simulink model "px4demo_mavlink_rc"  (R2017b)
settings: Solver=FixedStepDiscrete  StartTime=0.0  StopTime=inf  RelTol=1e-3  EnableMultiTasking=on
undefined symbols (not defined in the file or in its folder): RC_INPUT_SOURCE_ENUM, RGBLED_COLOR_ENUM, RGBLED_MODE_ENUM
libraries: pixhawk_slib_sensors_actuators x2, simulink x1, pixhawk_slib_uORB_RW x1
Description:
  | PX4 PSP Demo Model publishing a MAVLINK status text message
  | 
  | Example model for using MAVLINK in Simulink
settings Model: Creator=skuznick  LastModifiedBy=skuznick
settings SolverCC: PositivePriorityOrder=on
settings OptimizationCC: DefaultParameterBehavior=Inlined  PassReuseOutputArgsAs=Individual arguments  MaxStackSize=64
settings DebuggingCC: ParameterTunabilityLossMsg=error
settings HardwareCC: ProdBitPerPointer=32  ProdBitPerSizeT=32  ProdBitPerPtrDiffT=32  ProdLargestAtomicInteger=Long  ProdLargestAtomicFloat=Double  ProdWordSize=32  ProdHWDeviceType=ARM Compatible->ARM Cortex
settings SFSimCC: MATLABDynamicMemAlloc=off
settings RTWCC: SystemTargetFile=ert.tlc  HardwareBoard=Pixhawk PX4  TemplateMakefile=ert_default_tmf  GenerateReport=on  Toolchain=Pixhawk Toolchain  BuildConfiguration=Faster Runs  IncludeHyperlinkInReport=on  LaunchReport=on  GenerateTraceInfo=on  GenerateTraceReport=on  GenerateTraceReportSl=on  GenerateTraceReportSf=on  GenerateTraceReportEml=on
settings CodeAppCC: ForceParamTrailComments=on  IgnoreCustomStorageClasses=off  OperatorAnnotations=on  SimulinkDataObjDesc=on  SFDataObjDesc=on  MATLABFcnDesc=on  InsertBlockDesc=on  StateflowObjectComments=on  MATLABSourceComments=on
settings ERTTargetCC: InlinedParameterPlacement=NonHierarchical  ERTCustomFileTemplate=px4_codertarget_file_process.tlc

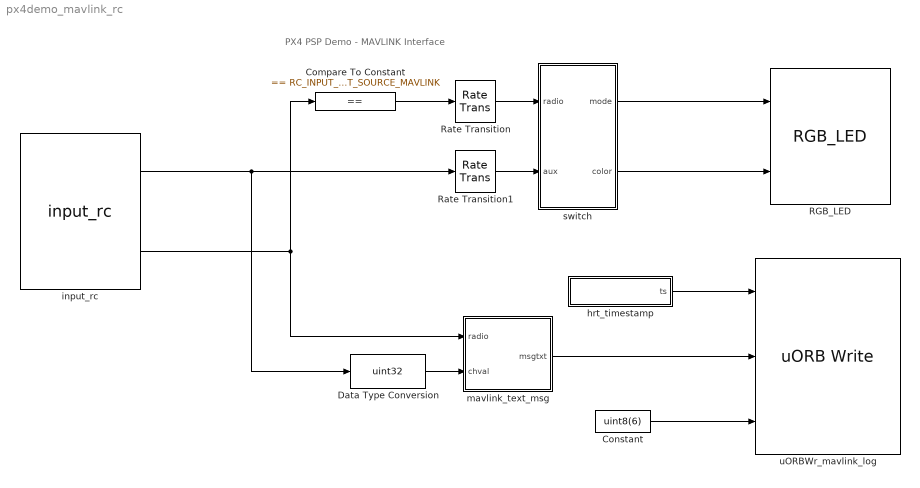
== system px4demo_mavlink_rc ==
  note: PX4 PSP Demo - MAVLINK Interface
  Compare To Constant : simulink/Logic and Bit Operations/Compare To Constant  relop===  const=RC_INPUT_SOURCE_ENUM.RCINPUT_SOURCE_MAVLINK  OutDataTypeStr=boolean
  Constant : Constant  Value=uint8(6)  SampleTime=-1
  Data Type Conversion : DataTypeConversion  OutDataTypeStr=uint32
  RGB_LED : pixhawk_slib_sensors_actuators/RGB_LED
      settings: SourceProductName=Pixhawk Target Blocks
  Rate Transition : RateTransition  OutPortSampleTime=1
  Rate Transition1 : RateTransition  OutPortSampleTime=1
  hrt_timestamp : MATLAB Function  TreatAsAtomicUnit=on
  input_rc : pixhawk_slib_sensors_actuators/input_rc  sampletime=1/250  channel1=off  channel2=off  channel3=off  channel4=on  channel5=off  channel6=off  channel7=off  channel8=off  channel9=off  channel10=off  channel11=off  channel12=off  channel13=off  channel14=off  channel15=off  channel16=off  channel17=off  channel18=off  ch_count=off  rssi=off  rc_failsafe=off  rc_lost=off  rc_inputsource=on
      settings: SourceProductName=Pixhawk Target Blocks
  mavlink_text_msg : MATLAB Function  TreatAsAtomicUnit=on
  switch : Subsystem
  uORBWr_mavlink_log : pixhawk_slib_uORB_RW/uORB Write  uORB_Topic_str='mavlink_log'  BlockOutputCount=3  OutputBoolean_1=on  uORB_Param_Name1='timestamp'  uORB_Param_Name_DT1=double  VectorScalar_1=1  OutputBoolean_2=on  uORB_Param_Name2='text'  uORB_Param_Name_DT2=uint8  VectorScalar_2=50  OutputBoolean_3=on  uORB_Param_Name3='severity'  uORB_Param_Name_DT3=uint8  VectorScalar_3=1  OutputBoolean_4=off  uORB_Param_Name4='gyro_temp'  uORB_Param_Name_DT4=single  VectorScalar_4=3  OutputBoolean_5=off  uORB_Param_Name5='vel_ned_valid'  uORB_Param_Name_DT5=boolean  VectorScalar_5=1  Ts=-1  MsgSizeOf=0
      settings: SourceProductName=Pixhawk Target Blocks
  wires:
  hrt_timestamp/1(ts) -> uORBWr_mavlink_log/1
  Compare To Constant/1 -> Rate Transition/1
  Constant/1 -> uORBWr_mavlink_log/3
  switch/1(mode) -> RGB_LED/1
  switch/2(color) -> RGB_LED/2
  Rate Transition/1 -> switch/1(radio)
  Rate Transition1/1 -> switch/2(aux)
  mavlink_text_msg/1(msgtxt) -> uORBWr_mavlink_log/2
  input_rc/1 -> Data Type Conversion/1, Rate Transition1/1
  input_rc/2 -> mavlink_text_msg/1(radio), Compare To Constant/1
  Data Type Conversion/1 -> mavlink_text_msg/2(chval)

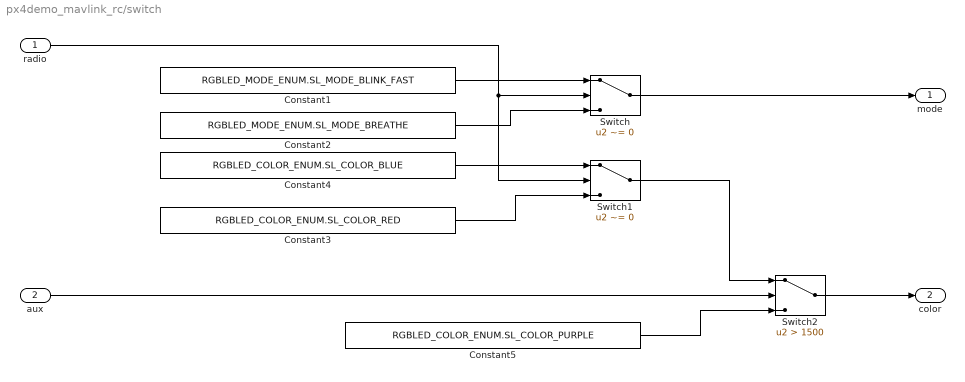
== system px4demo_mavlink_rc/switch ==
  radio : Inport
  aux : Inport  Port=2
  Constant1 : Constant  Value=RGBLED_MODE_ENUM.SL_MODE_BLINK_FAST  OutDataTypeStr=Enum: RGBLED_MODE_ENUM
  Constant2 : Constant  Value=RGBLED_MODE_ENUM.SL_MODE_BREATHE  OutDataTypeStr=Enum: RGBLED_MODE_ENUM
  Constant3 : Constant  Value=RGBLED_COLOR_ENUM.SL_COLOR_RED  OutDataTypeStr=Enum: RGBLED_COLOR_ENUM
  Constant4 : Constant  Value=RGBLED_COLOR_ENUM.SL_COLOR_BLUE  OutDataTypeStr=Enum: RGBLED_COLOR_ENUM
  Constant5 : Constant  Value=RGBLED_COLOR_ENUM.SL_COLOR_PURPLE  OutDataTypeStr=Enum: RGBLED_COLOR_ENUM
  Switch : Switch  Criteria=u2 ~= 0  Threshold=1500
  Switch1 : Switch  Criteria=u2 ~= 0  Threshold=1500
  Switch2 : Switch  Criteria=u2 > Threshold  Threshold=1500
  mode : Outport
  color : Outport  Port=2
  wires:
  Switch1/1 -> Switch2/1
  Constant5/1 -> Switch2/3
  Switch2/1 -> color/1
  aux/1 -> Switch2/2
  Switch/1 -> mode/1
  radio/1 -> Switch/2, Switch1/2
  Constant3/1 -> Switch1/3
  Constant1/1 -> Switch/1
  Constant2/1 -> Switch/3
  Constant4/1 -> Switch1/1

== matlab function px4demo_mavlink_rc/hrt_timestamp ==
  data: ts output
function ts  = fcn
% coder.cinclude('drivers/drv_hrt.h');
persistent count
if isempty(count)
    count = 0;
end

hrt = 0;
if coder.target('Rtw')
    hrt = coder.ceval('(double)hrt_absolute_time');
else
    hrt = count;
end
ts = hrt;

count = count + 1;

== matlab function px4demo_mavlink_rc/mavlink_text_msg ==
  data: msgtxt output; radio input; chval input
function msgtxt  = fcn(radio, chval)

% coder.cinclude('drivers/drv_hrt.h');

persistent count
if isempty(count)
    count = uint8('A');
end

msgtxt = zeros(1,50,'uint8');
coder.ceval('sprintf', coder.wref(msgtxt), 'Simulink [%c] Radio %d Value %d', count, int32(radio), int32(chval));

count = count + uint8(1);
if count == uint8('Z')
    count = uint8('A');
end
